simulink model "pendule_inv_etu"  (R2022a)
settings: Solver=VariableStepAuto  StartTime=0.0  StopTime=10.0  RelTol=1e-3
values from neighbouring files (symbols this model uses):
  g = 9.81    [simu_pendule_inv_capteur_etu.m]    (also in simu_pendule_inv_echant_etu.m; simu_pendule_inv_etu.m)
  K = [10 1]    [simu_pendule_inv_capteur_etu.m]    (also in simu_pendule_inv_echant_etu.m = [30 10]; simu_pendule_inv_etu.m = [30 10])
  l = 10    [simu_pendule_inv_capteur_etu.m]    (also in simu_pendule_inv_echant_etu.m; simu_pendule_inv_etu.m)
  ue = 0    [simu_pendule_inv_capteur_etu.m]    (also in simu_pendule_inv_echant_etu.m; simu_pendule_inv_etu.m)
  x0 = [pi/20 0]'    [simu_pendule_inv_capteur_etu.m]    (also in simu_pendule_inv_echant_etu.m; simu_pendule_inv_etu.m = [pi/10 0]')
  xe = [0 0]'    [simu_pendule_inv_capteur_etu.m]    (also in simu_pendule_inv_echant_etu.m; simu_pendule_inv_etu.m)
settings Model: Creator=nauchere  LastModifiedBy=nauchere

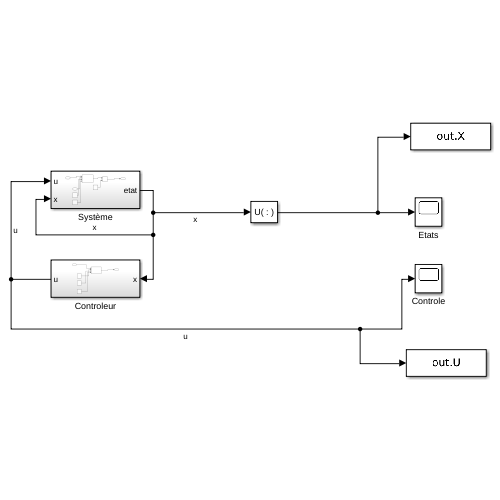
[thumbnail: Simulink's stored preview of the top-level diagram]
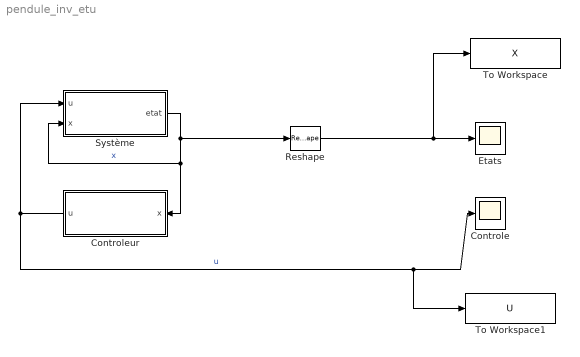
== system pendule_inv_etu ==
  Controle : Scope
  Controleur : Subsystem
  Etats : Scope
  Reshape : Reshape
  Système : Subsystem
  To Workspace : ToWorkspace  VariableName=X  SaveFormat=Timeseries  SampleTime=-1
  To Workspace1 : ToWorkspace  VariableName=U  SaveFormat=Timeseries  SampleTime=-1
  wires:
  Système/1(etat) -> Reshape/1, Système/2(x), Controleur/1(x)  "x"
  Controleur/1(u) -> Système/1(u), To Workspace1/1, Controle/1  "u"
  Reshape/1 -> To Workspace/1, Etats/1

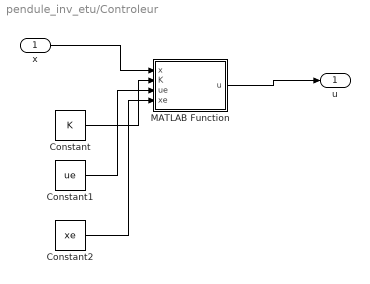
== system pendule_inv_etu/Controleur ==
  x : Inport
  Constant : Constant  Value=K  VectorParams1D=off
  Constant1 : Constant  Value=ue
  Constant2 : Constant  Value=xe  VectorParams1D=off
  MATLAB Function : MATLAB Function  TreatAsAtomicUnit=on
  u : Outport
  wires:
  x/1 -> MATLAB Function/1(x)
  MATLAB Function/1(u) -> u/1
  Constant/1 -> MATLAB Function/2(K)
  Constant1/1 -> MATLAB Function/3(ue)
  Constant2/1 -> MATLAB Function/4(xe)

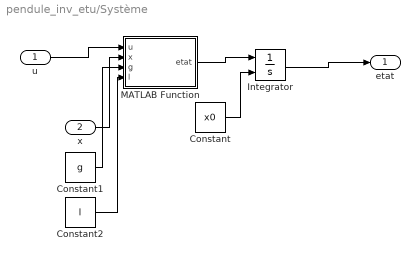
== system pendule_inv_etu/Système ==
  u : Inport
  x : Inport  Port=2
  Constant : Constant  Value=x0  VectorParams1D=off
  Constant1 : Constant  Value=g
  Constant2 : Constant  Value=l
  Integrator : Integrator  InitialConditionSource=external
  MATLAB Function : MATLAB Function  TreatAsAtomicUnit=on
  etat : Outport
  wires:
  u/1 -> MATLAB Function/1(u)
  x/1 -> MATLAB Function/2(x)
  Integrator/1 -> etat/1
  MATLAB Function/1(etat) -> Integrator/1
  Constant/1 -> Integrator/2
  Constant1/1 -> MATLAB Function/3(g)
  Constant2/1 -> MATLAB Function/4(l)

== matlab function pendule_inv_etu/Controleur/MATLAB Function ==
  data: x input; u output; K input; ue input; xe input
function u = fcn(x, K, ue, xe)

u = ue + K*(x - xe);
end

== matlab function pendule_inv_etu/Système/MATLAB Function ==
  data: u input; etat output; x input; g input; l input
function etat = fcn(u,x, g, l)
    x1_p = x(2);
    x2_p = (g/l)*sin(x(1)) - (cos(x(1))*u)/l;
etat = [x1_p x2_p]';
end
